simulink model "main"  (R2022a)
settings: Solver=FixedStepDiscrete  StartTime=0.0  StopTime=Inf  FixedStep=(50e-6)-(sim_en*4.995e-5)  RelTol=1e-3  EnableMultiTasking=on
model workspace (MAT data in the model file):
  Param : Simulink.Parameter (value not decoded)
  ac_ok : Simulink.Signal (value not decoded)
  ac_ok_120 : Simulink.Signal (value not decoded)
  bulk_voltage : Simulink.Signal (value not decoded)
  burstduty_integ_max : Simulink.Signal (value not decoded)
  burstduty_integ_min : Simulink.Signal (value not decoded)
  burstduty_ki : Simulink.Signal (value not decoded)
  burstduty_kp : Simulink.Signal (value not decoded)
  calib_ok : Simulink.Signal (value not decoded)
  can_addr1 : Simulink.Signal (value not decoded)
  can_addr2 : Simulink.Signal (value not decoded)
  can_addr3 : Simulink.Signal (value not decoded)
  can_addr4 : Simulink.Signal (value not decoded)
  can_data_rx : Simulink.Signal (value not decoded)
  can_data_tx : Simulink.Signal (value not decoded)
  can_timeout_120 : Simulink.Signal (value not decoded)
  chksum_scircv : Simulink.Signal (value not decoded)
  clllc_en_120 : Simulink.Signal (value not decoded)
  clllc_fault_120 : Simulink.Signal (value not decoded)
  clllc_ok_120 : Simulink.Signal (value not decoded)
  cmpss1h : Simulink.Signal (value not decoded)
  cmpss1l : Simulink.Signal (value not decoded)
  cmpss2h : Simulink.Signal (value not decoded)
  cmpss2l : Simulink.Signal (value not decoded)
  cmpss3h : Simulink.Signal (value not decoded)
  cmpss3l : Simulink.Signal (value not decoded)
  cmpss4h : Simulink.Signal (value not decoded)
  cmpss4l : Simulink.Signal (value not decoded)
  cmpss5h : Simulink.Signal (value not decoded)
  cmpss5l : Simulink.Signal (value not decoded)
  cmpss6h : Simulink.Signal (value not decoded)
  cmpss6l : Simulink.Signal (value not decoded)
  cmpss7h : Simulink.Signal (value not decoded)
  cmpss7l : Simulink.Signal (value not decoded)
  cmpss8h : Simulink.Signal (value not decoded)
  cmpss8l : Simulink.Signal (value not decoded)
  cnt_idle : Simulink.Signal (value not decoded)
  cnt_orps : Simulink.Signal (value not decoded)
  cnt_scircv : Simulink.Signal (value not decoded)
  cnt_scixmt : Simulink.Signal (value not decoded)
  cnt_scixmt_func : Simulink.Signal (value not decoded)
  cnt_temp_mux : Simulink.Signal (value not decoded)
  cnt_vdroop : Simulink.Signal (value not decoded)
  config_ok : Simulink.Signal (value not decoded)
  control_en : Simulink.Signal (value not decoded)
  cp_ready_120 : Simulink.Signal (value not decoded)
  d2d_en : Simulink.Signal (value not decoded)
  dchg_off : Simulink.Signal (value not decoded)
  debug_dacb : Simulink.Signal (value not decoded)
  debug_dacc : Simulink.Signal (value not decoded)
  debug_msg1 : Simulink.Signal (value not decoded)
  debug_msg2 : Simulink.Signal (value not decoded)
  debug_msg3 : Simulink.Signal (value not decoded)
  debug_msg4 : Simulink.Signal (value not decoded)
  debug_msg5 : Simulink.Signal (value not decoded)
  debug_msg6 : Simulink.Signal (value not decoded)
  dir_v2g : Simulink.Signal (value not decoded)
  eoss_llc1 : Simulink.Signal (value not decoded)
  eoss_llc2 : Simulink.Signal (value not decoded)
  eoss_orps : Simulink.Signal (value not decoded)
  fault_ocp : Simulink.Signal (value not decoded)
  fault_otp : Simulink.Signal (value not decoded)
  fault_ovp : Simulink.Signal (value not decoded)
  fut_en : Simulink.Signal (value not decoded)
  fwd_en_120 : Simulink.Signal (value not decoded)
  gain_llc1_sec_idc : Simulink.Signal (value not decoded)
  gain_llc1_temp_sr : Simulink.Signal (value not decoded)
  gain_llc2_sec_idc : Simulink.Signal (value not decoded)
  gain_vbat : Simulink.Signal (value not decoded)
  gain_vbulk : Simulink.Signal (value not decoded)
  gain_vout : Simulink.Signal (value not decoded)
  input_current_phasea : Simulink.Signal (value not decoded)
  input_current_phaseb : Simulink.Signal (value not decoded)
  input_current_phasec : Simulink.Signal (value not decoded)
  input_freq : Simulink.Signal (value not decoded)
  input_power : Simulink.Signal (value not decoded)
  input_voltage_phasea : Simulink.Signal (value not decoded)
  input_voltage_phaseb : Simulink.Signal (value not decoded)
  input_voltage_phasec : Simulink.Signal (value not decoded)
  ishare_arbiter : Simulink.Signal (value not decoded)
  ishare_thresh : Simulink.Signal (value not decoded)
  led_g : Simulink.Signal (value not decoded)
  led_r : Simulink.Signal (value not decoded)
  led_y : Simulink.Signal (value not decoded)
  llc1_burst_integ : Simulink.Signal (value not decoded)
  llc1_burstduty_buffer : Simulink.Signal (value not decoded)
  llc1_pfm_error : Simulink.Signal (value not decoded)
  llc1_pfm_integ : Simulink.Signal (value not decoded)
  llc1_pfm_prop : Simulink.Signal (value not decoded)
  llc1_pri_idc : Simulink.Signal (value not decoded)
  llc1_ps_buffer : Simulink.Signal (value not decoded)
  llc1_pspwm_error : Simulink.Signal (value not decoded)
  llc1_pspwm_integ : Simulink.Signal (value not decoded)
  llc1_pspwm_prop : Simulink.Signal (value not decoded)
  llc1_sec_idc : Simulink.Signal (value not decoded)
  llc1_temp_sr : Simulink.Signal (value not decoded)
  llc1_ts_tbctr_buffer : Simulink.Signal (value not decoded)
  llc2_burst_integ : Simulink.Signal (value not decoded)
  llc2_burstduty_buffer : Simulink.Signal (value not decoded)
  llc2_en : Simulink.Signal (value not decoded)
  llc2_en_buffer : Simulink.Signal (value not decoded)
  llc2_pfm_error : Simulink.Signal (value not decoded)
  llc2_pfm_integ : Simulink.Signal (value not decoded)
  llc2_pfm_prop : Simulink.Signal (value not decoded)
  llc2_pri_idc : Simulink.Signal (value not decoded)
  llc2_ps_buffer : Simulink.Signal (value not decoded)
  llc2_pspwm_error : Simulink.Signal (value not decoded)
  llc2_pspwm_integ : Simulink.Signal (value not decoded)
  llc2_pspwm_prop : Simulink.Signal (value not decoded)
  llc2_sec_idc : Simulink.Signal (value not decoded)
  llc2_temp_sr : Simulink.Signal (value not decoded)
  llc2_ts_tbctr_buffer : Simulink.Signal (value not decoded)
  loop_adcint : Simulink.Signal (value not decoded)
  loop_control : Simulink.Signal (value not decoded)
  loop_idle : Simulink.Signal (value not decoded)
  mid_bulk_voltage : Simulink.Signal (value not decoded)
  mode_120 : Simulink.Signal (value not decoded)
  mode_cc_cv : Simulink.Signal (value not decoded)
  myParam : mpt.Parameter (value not decoded)
  obc_ok_120 : Simulink.Signal (value not decoded)
  offset_llc1_sec_idc : Simulink.Signal (value not decoded)
  offset_llc1_temp_sr : Simulink.Signal (value not decoded)
  offset_llc2_sec_idc : Simulink.Signal (value not decoded)
  offset_vbat : Simulink.Signal (value not decoded)
  offset_vbulk : Simulink.Signal (value not decoded)
  offset_vout : Simulink.Signal (value not decoded)
  openloop_en : Simulink.Signal (value not decoded)
  openloop_fault_en : Simulink.Signal (value not decoded)
  ot_fault_120 : Simulink.Signal (value not decoded)
  pfc_en : Simulink.Signal (value not decoded)
  pfc_en_120 : Simulink.Signal (value not decoded)
  pfc_fw_revision : Simulink.Signal (value not decoded)
  pfc_fw_revision_bootloader : Simulink.Signal (value not decoded)
  pfc_fw_revision_debug : Simulink.Signal (value not decoded)
  pfc_ok : Simulink.Signal (value not decoded)
  pfc_ok_120 : Simulink.Signal (value not decoded)
  pfm_a0 : Simulink.Signal (value not decoded)
  pfm_a1 : Simulink.Signal (value not decoded)
  pfm_integ_max : Simulink.Signal (value not decoded)
  pfm_integ_min : Simulink.Signal (value not decoded)
  pfm_ki : Simulink.Signal (value not decoded)
  pfm_kp : Simulink.Signal (value not decoded)
  pri_fut_en : Simulink.Signal (value not decoded)
  pri_fut_en_buffer : Simulink.Signal (value not decoded)
  pri_halfbridge_en : Simulink.Signal (value not decoded)
  pri_halfbridge_en_buffer : Simulink.Signal (value not decoded)
  pspwm_integ_max : Simulink.Signal (value not decoded)
  pspwm_integ_min : Simulink.Signal (value not decoded)
  pspwm_ki : Simulink.Signal (value not decoded)
  pspwm_kp : Simulink.Signal (value not decoded)
  ref_idclink_max : Simulink.Signal (value not decoded)
  ref_iout : Simulink.Signal (value not decoded)
  ref_iout_calib : Simulink.Signal (value not decoded)
  ref_iout_llc1 : Simulink.Signal (value not decoded)
  ref_iout_llc1_calib : Simulink.Signal (value not decoded)
  ref_iout_llc2 : Simulink.Signal (value not decoded)
  ref_iout_llc2_calib : Simulink.Signal (value not decoded)
  ref_pout : Simulink.Signal (value not decoded)
  ref_ss_llc1 : Simulink.Signal (value not decoded)
  ref_ss_llc2 : Simulink.Signal (value not decoded)
  ref_ss_orps : Simulink.Signal (value not decoded)
  ref_vbat : Simulink.Signal (value not decoded)
  ref_vbat_calib : Simulink.Signal (value not decoded)
  ref_vbulk : Simulink.Signal (value not decoded)
  ref_vbulk_calib : Simulink.Signal (value not decoded)
  ref_vbulk_llc1_calib : Simulink.Signal (value not decoded)
  ref_vbulk_llc2_calib : Simulink.Signal (value not decoded)
  ref_vout : Simulink.Signal (value not decoded)
  ref_vout_calib : Simulink.Signal (value not decoded)
  relay_en : Simulink.Signal (value not decoded)
  reset_flag : Simulink.Signal (value not decoded)
  rev_en_120 : Simulink.Signal (value not decoded)
  runtime_control : Simulink.Signal (value not decoded)
  runtime_idle : Simulink.Signal (value not decoded)
  scircv_buffer : Simulink.Signal (value not decoded)
  scircv_buffer_tmp : Simulink.Signal (value not decoded)
  scircv_buffer_tmp_idx0 : Simulink.Signal (value not decoded)
  scircv_chksum : Simulink.Signal (value not decoded)
  scircv_chksum_ok : Simulink.Signal (value not decoded)
  scircv_parse_ok : Simulink.Signal (value not decoded)
  scixmt_buffer : Simulink.Signal (value not decoded)
  scixmt_chksum : Simulink.Signal (value not decoded)
  scixmt_func : Simulink.Signal (value not decoded)
  scixmt_word0_lsb : Simulink.Signal (value not decoded)
  scixmt_word0_msb : Simulink.Signal (value not decoded)
  scixmt_word1_lsb : Simulink.Signal (value not decoded)
  scixmt_word1_msb : Simulink.Signal (value not decoded)
  scixmt_word2_lsb : Simulink.Signal (value not decoded)
  scixmt_word2_msb : Simulink.Signal (value not decoded)
  scixmt_wr : Simulink.Signal (value not decoded)
  ss_step : Simulink.Signal (value not decoded)
  state_calib : Simulink.Signal (value not decoded)
  state_control : Simulink.Signal (value not decoded)
  state_hkeep : Simulink.Signal (value not decoded)
  status_cmpss : Simulink.Signal (value not decoded)
  status_control : Simulink.Signal (value not decoded)
  status_digin : Simulink.Signal (value not decoded)
  status_digout : Simulink.Signal (value not decoded)
  status_fault : Simulink.Signal (value not decoded)
  status_input : Simulink.Signal (value not decoded)
  status_pfc : Simulink.Signal (value not decoded)
  temp_inlet : Simulink.Signal (value not decoded)
  temp_llc1_fet_hs : Simulink.Signal (value not decoded)
  temp_llc2_fet_hs : Simulink.Signal (value not decoded)
  temp_mux : Simulink.Signal (value not decoded)
  temp_mux_s0 : Simulink.Signal (value not decoded)
  temp_mux_s1 : Simulink.Signal (value not decoded)
  temp_mux_s2 : Simulink.Signal (value not decoded)
  temp_outlet : Simulink.Signal (value not decoded)
  temp_pfc_fet_hsa : Simulink.Signal (value not decoded)
  temp_pfc_fet_hsb : Simulink.Signal (value not decoded)
  temp_pfc_fet_hsc : Simulink.Signal (value not decoded)
  temp_pfc_fet_lsa : Simulink.Signal (value not decoded)
  temp_pfc_fet_lsb : Simulink.Signal (value not decoded)
  temp_pfc_fet_lsc : Simulink.Signal (value not decoded)
  test_mode : Simulink.Signal (value not decoded)
  tfcv_cc : Simulink.Signal (value not decoded)
  tfcv_cc_llc2 : Simulink.Signal (value not decoded)
  tfcv_cv : Simulink.Signal (value not decoded)
  tfcv_sr_en : Simulink.Signal (value not decoded)
  tfv_assert_llc1_pri_idc : Simulink.Signal (value not decoded)
  tfv_assert_llc1_sec_idc : Simulink.Signal (value not decoded)
  tfv_assert_llc1_temp_sr : Simulink.Signal (value not decoded)
  tfv_assert_llc2_pri_idc : Simulink.Signal (value not decoded)
  tfv_assert_llc2_sec_idc : Simulink.Signal (value not decoded)
  tfv_assert_llc2_temp_sr : Simulink.Signal (value not decoded)
  tfv_assert_temp_outlet : Simulink.Signal (value not decoded)
  tfv_assert_vaux_uv : Simulink.Signal (value not decoded)
  tfv_assert_vbat : Simulink.Signal (value not decoded)
  tfv_assert_vbulk : Simulink.Signal (value not decoded)
  tfv_assert_vout : Simulink.Signal (value not decoded)
  tfv_cnt_tz : Simulink.Signal (value not decoded)
  tfv_deassert_llc1_pri_idc : Simulink.Signal (value not decoded)
  tfv_deassert_llc1_sec_idc : Simulink.Signal (value not decoded)
  tfv_deassert_llc1_temp_sr : Simulink.Signal (value not decoded)
  tfv_deassert_llc2_pri_idc : Simulink.Signal (value not decoded)
  tfv_deassert_llc2_sec_idc : Simulink.Signal (value not decoded)
  tfv_deassert_llc2_temp_sr : Simulink.Signal (value not decoded)
  tfv_deassert_temp_outlet : Simulink.Signal (value not decoded)
  tfv_deassert_vaux_uv : Simulink.Signal (value not decoded)
  tfv_deassert_vbat : Simulink.Signal (value not decoded)
  tfv_deassert_vbulk : Simulink.Signal (value not decoded)
  tfv_deassert_vout : Simulink.Signal (value not decoded)
  tfv_llc1_pri_idc : Simulink.Signal (value not decoded)
  tfv_llc1_sec_idc : Simulink.Signal (value not decoded)
  tfv_llc1_temp_sr : Simulink.Signal (value not decoded)
  tfv_llc2_pri_idc : Simulink.Signal (value not decoded)
  tfv_llc2_sec_idc : Simulink.Signal (value not decoded)
  tfv_llc2_temp_sr : Simulink.Signal (value not decoded)
  tfv_temp_outlet : Simulink.Signal (value not decoded)
  tfv_vaux_uv : Simulink.Signal (value not decoded)
  tfv_vbat : Simulink.Signal (value not decoded)
  tfv_vbulk : Simulink.Signal (value not decoded)
  tfv_vout : Simulink.Signal (value not decoded)
  timer_1ms : Simulink.Signal (value not decoded)
  tz : Simulink.Signal (value not decoded)
  valve_en : Simulink.Signal (value not decoded)
  vaux : Simulink.Signal (value not decoded)
  vbat : Simulink.Signal (value not decoded)
  vbulk : Simulink.Signal (value not decoded)
  vout : Simulink.Signal (value not decoded)
undefined symbols (not defined in the file or in its folder): CAN_O_INT, CANA_BASE, Down, GPTRIP1SEL, GPTRIP2SEL, TZ1, TZ2, Up
libraries: hdlsllib x159, simulink x100, c2837xDlib x24, c2807xlib x16, c280xlib x13, c2802xlib x12, canmsglib x8, idelinklib_common x2, c2000lib x1, c281xlib x1
(part 8 of 15)

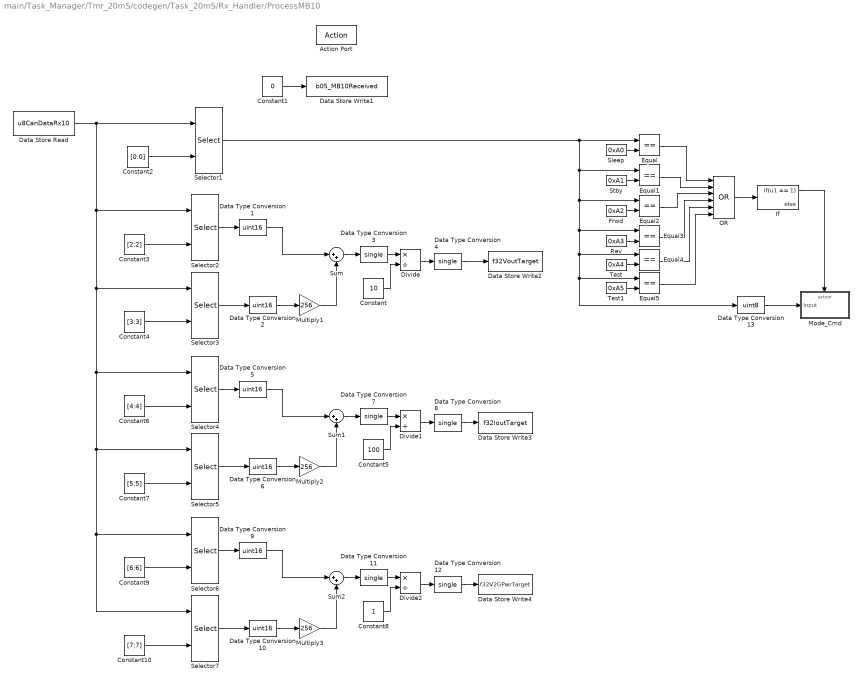
== system main/Task_Manager/Tmr_20mS/codegen/Task_20mS/Rx_Handler/ProcessMB10 ==
  Action Port : ActionPort  ActionPortLabel=if(u1 == 1)
  Constant : Constant  Value=10
  Constant1 : Constant  Value=0  OutDataTypeStr=boolean
  Constant10 : Constant  Value=[7:7]
  Constant2 : Constant  Value=[0:0]
  Constant3 : Constant  Value=[2:2]
  Constant4 : Constant  Value=[3:3]
  Constant5 : Constant  Value=100
  Constant6 : Constant  Value=[4:4]
  Constant7 : Constant  Value=[5:5]
  Constant8 : Constant
  Constant9 : Constant  Value=[6:6]
  Data Store Read : DataStoreRead  DataStoreName=u8CanDataRx10  IndexOptions=Index vector (dialog)  Indices=1  OutputSizes=1
  Data Store Write1 : DataStoreWrite  DataStoreName=b05_MB10Received  IndexOptions=Index vector (dialog)  Indices=1  OutputSizes=1
  Data Store Write2 : DataStoreWrite  DataStoreName=f32VoutTarget  IndexOptions=Index vector (dialog)  Indices=1  OutputSizes=1
  Data Store Write3 : DataStoreWrite  DataStoreName=f32IoutTarget  IndexOptions=Index vector (dialog)  Indices=1  OutputSizes=1
  Data Store Write4 : DataStoreWrite  DataStoreName=f32V2GPwrTarget  IndexOptions=Index vector (dialog)  Indices=1  OutputSizes=1
  Data Type Conversion{1..2,5..6,9..10} (6 alike) : DataTypeConversion  OutDataTypeStr=uint16  SaturateOnIntegerOverflow=off  RndMeth=Floor
  Data Type Conversion{3..4,7..8,11..12} (6 alike) : DataTypeConversion  OutDataTypeStr=single  SaturateOnIntegerOverflow=off  RndMeth=Floor
  Data Type Conversion13 : DataTypeConversion  OutDataTypeStr=uint8  SaturateOnIntegerOverflow=off  RndMeth=Floor
  Divide : Product  Inputs=*/
  Divide1 : Product  Inputs=*/
  Divide2 : Product  Inputs=*/
  Equal{,1..5} (6 alike) : RelationalOperator  Operator===  OutDataTypeStr=boolean  RndMeth=Simplest  InputSameDT=off
  Frwd : Constant  Value=0xA2
  If : If  IfExpression=u1 == 1
  Mode_Cmd : Subsystem  TreatAsAtomicUnit=on
  Multiply1 : Gain  Gain=256
  Multiply2 : Gain  Gain=256
  Multiply3 : Gain  Gain=256
  OR : Logic  Operator=OR  Inputs=6  IconShape=distinctive  AllPortsSameDT=off  OutDataTypeStr=boolean
  Rev : Constant  Value=0xA3
  Selector{1..7} (7 alike) : Selector  IndexMode=Zero-based  InputPortWidth=8  IndexOptions=Index vector (port)  Indices=[1 3]  OutputSizes=1
  Sleep : Constant  Value=0xA0
  Stby : Constant  Value=0xA1
  Sum : Sum  Inputs=|++
  Sum1 : Sum  Inputs=|++
  Sum2 : Sum  Inputs=|++
  Test : Constant  Value=0xA4
  Test1 : Constant  Value=0xA5
  wires:
  Constant1/1 -> Data Store Write1/1
  Constant2/1 -> Selector1/2
  Constant3/1 -> Selector2/2
  Constant4/1 -> Selector3/2
  Selector2/1 -> Data Type Conversion1/1
  Data Type Conversion1/1 -> Sum/1
  Selector3/1 -> Data Type Conversion2/1
  Data Type Conversion2/1 -> Multiply1/1
  Multiply1/1 -> Sum/2
  Sum/1 -> Data Type Conversion3/1
  Constant/1 -> Divide/2
  Divide/1 -> Data Type Conversion4/1
  Data Type Conversion3/1 -> Divide/1
  Data Type Conversion4/1 -> Data Store Write2/1
  Data Type Conversion8/1 -> Data Store Write3/1
  Data Type Conversion7/1 -> Divide1/1
  Divide1/1 -> Data Type Conversion8/1
  Constant5/1 -> Divide1/2
  Sum1/1 -> Data Type Conversion7/1
  Multiply2/1 -> Sum1/2
  Data Type Conversion6/1 -> Multiply2/1
  Selector5/1 -> Data Type Conversion6/1
  Data Type Conversion5/1 -> Sum1/1
  Selector4/1 -> Data Type Conversion5/1
  Constant7/1 -> Selector5/2
  Constant6/1 -> Selector4/2
  Constant9/1 -> Selector6/2
  Data Store Read/1 -> Selector6/1, Selector7/1, Selector5/1, Selector4/1, Selector3/1, Selector2/1, Selector1/1
  Constant10/1 -> Selector7/2
  Selector6/1 -> Data Type Conversion9/1
  Data Type Conversion9/1 -> Sum2/1
  Selector7/1 -> Data Type Conversion10/1
  Data Type Conversion10/1 -> Multiply3/1
  Multiply3/1 -> Sum2/2
  Sum2/1 -> Data Type Conversion11/1
  Constant8/1 -> Divide2/2
  Divide2/1 -> Data Type Conversion12/1
  Data Type Conversion11/1 -> Divide2/1
  Data Type Conversion12/1 -> Data Store Write4/1
  Stby/1 -> Equal1/2
  OR/1 -> If/1
  Rev/1 -> Equal3/2
  Equal1/1 -> OR/2
  Frwd/1 -> Equal2/2
  Equal2/1 -> OR/3
  Equal3/1 -> OR/4
  Data Type Conversion13/1 -> Mode_Cmd/1(Input)
  Equal/1 -> OR/1
  Sleep/1 -> Equal/2
  If/1 -> Mode_Cmd/Action
  Equal4/1 -> OR/5
  Selector1/1 -> Equal4/1, Data Type Conversion13/1, Equal5/1, Equal3/1, Equal2/1, Equal1/1, Equal/1
  Test/1 -> Equal4/2
  Equal5/1 -> OR/6
  Test1/1 -> Equal5/2

== system main/Task_Manager/Tmr_20mS/codegen/Task_20mS/Rx_Handler/ProcessMB11 ==
  Action Port : ActionPort  ActionPortLabel=elseif(u2 ==1)
  Constant : Constant  Value=0  OutDataTypeStr=boolean
  Constant1 : Constant  Value=[1:1]
  Constant2 : Constant  Value=[0:0]
  Data Store Read : DataStoreRead  DataStoreName=u8CanDataRx11  IndexOptions=Index vector (dialog)  Indices=1  OutputSizes=1
  Data Store Write1 : DataStoreWrite  DataStoreName=b06_MB11Received  IndexOptions=Index vector (dialog)  Indices=1  OutputSizes=1
  Data Store Write5 : DataStoreWrite  DataStoreName=u8AliveCounter  IndexOptions=Index vector (dialog)  Indices=1  OutputSizes=1
  Data Type Conversion : DataTypeConversion  OutDataTypeStr=uint8  SaturateOnIntegerOverflow=off  RndMeth=Floor
  Data Type Conversion1 : DataTypeConversion  OutDataTypeStr=uint8  SaturateOnIntegerOverflow=off  RndMeth=Floor
  Equal{,1..3} (4 alike) : RelationalOperator  Operator===  OutDataTypeStr=boolean  RndMeth=Simplest  InputSameDT=off
  If : If  IfExpression=u1 == 1
  OR : Logic  Operator=OR  Inputs=4  IconShape=distinctive  AllPortsSameDT=off  OutDataTypeStr=boolean
  Red_Frwd : Constant  Value=0xB2
  Red_Mode_Cmd : Subsystem  TreatAsAtomicUnit=on
  Red_Rev : Constant  Value=0xB3
  Red_Sleep : Constant  Value=0xB0
  Red_Stby : Constant  Value=0xB1
  Selector1 : Selector  IndexMode=Zero-based  InputPortWidth=8  IndexOptions=Index vector (port)  Indices=[1 3]  OutputSizes=1
  Selector2 : Selector  IndexMode=Zero-based  InputPortWidth=8  IndexOptions=Index vector (port)  Indices=[1 3]  OutputSizes=1
  wires:
  Constant/1 -> Data Store Write1/1
  Constant2/1 -> Selector1/2
  Data Type Conversion/1 -> Data Store Write5/1
  Selector1/1 -> Data Type Conversion/1
  Data Store Read/1 -> Selector2/1, Selector1/1
  Constant1/1 -> Selector2/2
  Red_Stby/1 -> Equal1/2
  Selector2/1 -> Equal/1, Data Type Conversion1/1, Equal3/1, Equal2/1, Equal1/1
  Equal2/1 -> OR/3
  Equal/1 -> OR/1
  If/1 -> Red_Mode_Cmd/Action
  OR/1 -> If/1
  Equal3/1 -> OR/4
  Equal1/1 -> OR/2
  Red_Rev/1 -> Equal3/2
  Red_Sleep/1 -> Equal/2
  Red_Frwd/1 -> Equal2/2
  Data Type Conversion1/1 -> Red_Mode_Cmd/1(Input)

== system main/Task_Manager/Tmr_20mS/codegen/Task_20mS/Rx_Handler/ProcessMB12 ==
  Action Port : ActionPort  ActionPortLabel=elseif( u3==1)
  Constant : Constant  Value=0  OutDataTypeStr=boolean
  Constant2 : Constant  Value=[0:0]
  Data Store Read : DataStoreRead  DataStoreName=u8CanDataRx12  IndexOptions=Index vector (dialog)  Indices=1  OutputSizes=1
  Data Store Write1 : DataStoreWrite  DataStoreName=b07_MB12Received  IndexOptions=Index vector (dialog)  Indices=1  OutputSizes=1
  Debug_Cmd : Subsystem  TreatAsAtomicUnit=on
  Debug_Read : Subsystem  TreatAsAtomicUnit=on
  Debug_Write : Subsystem  TreatAsAtomicUnit=on
  If : If  IfExpression=u1 == 0  ElseIfExpressions=u1 ==1, u1==2
  Selector1 : Selector  IndexMode=Zero-based  InputPortWidth=8  IndexOptions=Index vector (port)  Indices=[1 3]  OutputSizes=1
  wires:
  Constant/1 -> Data Store Write1/1
  Constant2/1 -> Selector1/2
  Data Store Read/1 -> Selector1/1
  Selector1/1 -> If/1
  If/1 -> Debug_Read/Action
  If/2 -> Debug_Write/Action
  If/3 -> Debug_Cmd/Action

== system main/Task_Manager/Tmr_20mS/codegen/Task_20mS/Tx_Handler/Run Tx Routine ==
  Action Port : ActionPort  ActionPortLabel=if(u1 == u2)
  Constant1 : Constant  Value=0  OutDataTypeStr=uint16
  Data Store Read2 : DataStoreRead  DataStoreName=b01_ReadRequest  IndexOptions=Index vector (dialog)  Indices=1  OutputSizes=1
  Data Store Read3 : DataStoreRead  DataStoreName=b00_DebugEnabled  IndexOptions=Index vector (dialog)  Indices=1  OutputSizes=1
  Data Store Write1 : DataStoreWrite  DataStoreName=u16TxDelayCount  IndexOptions=Index vector (dialog)  Indices=1  OutputSizes=1
  If1 : If  NumInputs=2  IfExpression=u1 == 1 & u2 == 1
  TxReadRequest : Subsystem  TreatAsAtomicUnit=on
  TxStatusData : Subsystem  TreatAsAtomicUnit=on
  wires:
  Constant1/1 -> Data Store Write1/1
  If1/1 -> TxReadRequest/Action
  If1/2 -> TxStatusData/Action
  Data Store Read3/1 -> If1/2
  Data Store Read2/1 -> If1/1

== system main/Task_Manager/idle/idle_task/comm_npc/comm_npc/COMM_NPC.calcScircvChksum/For Iterator Subsystem ==
  scircv_buffer : Inport
  Bitwise XOR : simulink/Logic and Bit Operations/Bitwise Operator  logicop=XOR  UseBitMask=off  NumInputPorts=2  BitMask=bin2dec('11011001')  BitMaskRealWorld=Stored Integer
  Data Store Read1 : DataStoreRead  DataStoreName=scircv_chksum  IndexOptions=Index vector (dialog)  Indices=1  OutputSizes=1
  Data Store Write : DataStoreWrite  DataStoreName=scircv_chksum  IndexOptions=Index vector (dialog)  Indices=1  OutputSizes=1
  For Iterator : ForIterator  IterationLimit=9  IndexMode=Zero-based  IterationVariableDataType=uint8
  Selector : Selector  IndexMode=Zero-based  InputPortWidth=12  IndexOptions=Index vector (port)  Indices=[1 3]  OutputSizes=1
  wires:
  For Iterator/1 -> Selector/2
  scircv_buffer/1 -> Selector/1
  Selector/1 -> Bitwise XOR/1
  Data Store Read1/1 -> Bitwise XOR/2
  Bitwise XOR/1 -> Data Store Write/1

== system main/Task_Manager/idle/idle_task/comm_npc/comm_npc/COMM_NPC.calcScixmtChksum/calc_chksum ==
  function : TriggerPort  TriggerType=function-call  VariantControl=Variant
  Data Store Read8 : DataStoreRead  DataStoreName=scixmt_buffer  IndexOptions=Index vector (dialog)  Indices=1  OutputSizes=1
  For Iterator Subsystem : Subsystem  TreatAsAtomicUnit=on
  wires:
  Data Store Read8/1 -> For Iterator Subsystem/1(scixmt_buffer)

== system main/Task_Manager/idle/idle_task/comm_npc/comm_npc/COMM_NPC.calcScixmtChksum/update_scixmt_buffer ==
  function : TriggerPort  TriggerType=function-call  VariantControl=Variant
  Data Store Read21 : DataStoreRead  DataStoreName=scixmt_func  IndexOptions=Index vector (dialog)  Indices=1  OutputSizes=1
  If : If  IfExpression=u1 == 33
  default : Subsystem  TreatAsAtomicUnit=on
  pri_fut_en : Subsystem  TreatAsAtomicUnit=on
  wires:
  If/1 -> pri_fut_en/Action
  If/2 -> default/Action
  Data Store Read21/1 -> default/1(scixmt_func), If/1

== system main/Task_Manager/idle/idle_task/comm_npc/comm_npc/COMM_NPC.extractScircv/input_main_info ==
  note: Note:
      | byte0 - header
      | byte1 - w/r
      | byte2 - func
      | byte3, byte4 - word0_lsb, word0_msb
      | byte5, byte6 - word1_lsb, word1_msb
      | byte7, byte8 - word2_lsb, word2_msb
      | byte9 - chksum
      | byte10 - 0x00
      | byte11 - terminator
  scircv_buffer : Inport
  Action Port : ActionPort  ActionPortLabel=case [ 1 ]:
  Add : Sum  AccumDataTypeStr=uint16  OutDataTypeStr=uint16
  Add1 : Sum  AccumDataTypeStr=uint16  OutDataTypeStr=uint16
  Add2 : Sum  AccumDataTypeStr=uint16  OutDataTypeStr=uint16
  Bit Shift : hdlsllib/Logic and Bit Operations/Bit Shift  mode=Shift Left Logical  N=8
  Bit Shift1 : hdlsllib/Logic and Bit Operations/Bit Shift  mode=Shift Left Logical  N=8
  Bit Shift2 : hdlsllib/Logic and Bit Operations/Bit Shift  mode=Shift Left Logical  N=8
  Cast To Single{1..6} (6 alike) : DataTypeConversion  OutDataTypeStr=uint16  SaturateOnIntegerOverflow=off  RndMeth=Floor
  Constant1 : Constant  Value=3  OutDataTypeStr=uint8
  Constant2 : Constant  Value=4  OutDataTypeStr=uint8
  Constant3 : Constant  Value=7  OutDataTypeStr=uint8
  Constant4 : Constant  Value=8  OutDataTypeStr=uint8
  Constant5 : Constant  Value=5  OutDataTypeStr=uint8
  Constant6 : Constant  Value=6  OutDataTypeStr=uint8
  Data Store Write1 : DataStoreWrite  DataStoreName=status_input  IndexOptions=Index vector (dialog)  Indices=1  OutputSizes=1
  Data Store Write2 : DataStoreWrite  DataStoreName=input_power  IndexOptions=Index vector (dialog)  Indices=1  OutputSizes=1
  Data Store Write3 : DataStoreWrite  DataStoreName=input_freq  IndexOptions=Index vector (dialog)  Indices=1  OutputSizes=1
  word0_lsb : Selector  IndexMode=Zero-based  InputPortWidth=12  IndexOptions=Index vector (port)  Indices=[1 3]  OutputSizes=1
  word0_lsb1 : Selector  IndexMode=Zero-based  InputPortWidth=12  IndexOptions=Index vector (port)  Indices=[1 3]  OutputSizes=1
  word0_lsb2 : Selector  IndexMode=Zero-based  InputPortWidth=12  IndexOptions=Index vector (port)  Indices=[1 3]  OutputSizes=1
  word0_msb : Selector  IndexMode=Zero-based  InputPortWidth=12  IndexOptions=Index vector (port)  Indices=[1 3]  OutputSizes=1
  word0_msb1 : Selector  IndexMode=Zero-based  InputPortWidth=12  IndexOptions=Index vector (port)  Indices=[1 3]  OutputSizes=1
  word0_msb2 : Selector  IndexMode=Zero-based  InputPortWidth=12  IndexOptions=Index vector (port)  Indices=[1 3]  OutputSizes=1
  wires:
  [scircv_buffer] -> word0_lsb2/1
  Constant5/1 -> word0_lsb2/2
  word0_lsb2/1 -> Cast To Single5/1
  Constant6/1 -> word0_msb2/2
  [scircv_buffer] -> word0_msb2/1
  word0_msb2/1 -> Cast To Single6/1
  Bit Shift2/1 -> Add2/2
  Add2/1 -> Data Store Write3/1
  Cast To Single5/1 -> Add2/1
  Cast To Single6/1 -> Bit Shift2/1
  [scircv_buffer] -> word0_lsb1/1
  Constant3/1 -> word0_lsb1/2
  word0_lsb1/1 -> Cast To Single3/1
  Constant4/1 -> word0_msb1/2
  [scircv_buffer] -> word0_msb1/1
  word0_msb1/1 -> Cast To Single4/1
  Bit Shift1/1 -> Add1/2
  Add1/1 -> Data Store Write2/1
  Cast To Single3/1 -> Add1/1
  Cast To Single4/1 -> Bit Shift1/1
  Cast To Single2/1 -> Bit Shift/1
  Cast To Single1/1 -> Add/1
  Add/1 -> Data Store Write1/1
  Bit Shift/1 -> Add/2
  word0_msb/1 -> Cast To Single2/1
  [scircv_buffer] -> word0_msb/1
  Constant2/1 -> word0_msb/2
  scircv_buffer/1 -> [scircv_buffer]
  word0_lsb/1 -> Cast To Single1/1
  Constant1/1 -> word0_lsb/2
  [scircv_buffer] -> word0_lsb/1

== system main/Task_Manager/idle/idle_task/comm_npc/comm_npc/COMM_NPC.extractScircv/input_phase_current ==
  note: Note:
      | byte0 - header
      | byte1 - w/r
      | byte2 - func
      | byte3, byte4 - word0_lsb, word0_msb
      | byte5, byte6 - word1_lsb, word1_msb
      | byte7, byte8 - word2_lsb, word2_msb
      | byte9 - chksum
      | byte10 - 0x00
      | byte11 - terminator
  scircv_buffer : Inport
  Action Port : ActionPort  ActionPortLabel=case [ 3 ]:
  Add : Sum  AccumDataTypeStr=uint16  OutDataTypeStr=uint16
  Add1 : Sum  AccumDataTypeStr=uint16  OutDataTypeStr=uint16
  Add2 : Sum  AccumDataTypeStr=uint16  OutDataTypeStr=uint16
  Bit Shift : hdlsllib/Logic and Bit Operations/Bit Shift  mode=Shift Left Logical  N=8
  Bit Shift1 : hdlsllib/Logic and Bit Operations/Bit Shift  mode=Shift Left Logical  N=8
  Bit Shift2 : hdlsllib/Logic and Bit Operations/Bit Shift  mode=Shift Left Logical  N=8
  Cast To Single{1..6} (6 alike) : DataTypeConversion  OutDataTypeStr=uint16  SaturateOnIntegerOverflow=off  RndMeth=Floor
  Constant1 : Constant  Value=3  OutDataTypeStr=uint8
  Constant2 : Constant  Value=4  OutDataTypeStr=uint8
  Constant3 : Constant  Value=7  OutDataTypeStr=uint8
  Constant4 : Constant  Value=8  OutDataTypeStr=uint8
  Constant5 : Constant  Value=5  OutDataTypeStr=uint8
  Constant6 : Constant  Value=6  OutDataTypeStr=uint8
  Data Store Write : DataStoreWrite  DataStoreName=input_current_phasea  IndexOptions=Index vector (dialog)  Indices=1  OutputSizes=1
  Data Store Write1 : DataStoreWrite  DataStoreName=input_current_phasea  IndexOptions=Index vector (dialog)  Indices=1  OutputSizes=1
  Data Store Write2 : DataStoreWrite  DataStoreName=input_current_phasec  IndexOptions=Index vector (dialog)  Indices=1  OutputSizes=1
  Data Store Write3 : DataStoreWrite  DataStoreName=input_current_phaseb  IndexOptions=Index vector (dialog)  Indices=1  OutputSizes=1
  Data Store Write4 : DataStoreWrite  DataStoreName=input_current_phaseb  IndexOptions=Index vector (dialog)  Indices=1  OutputSizes=1
  word0_lsb : Selector  IndexMode=Zero-based  InputPortWidth=12  IndexOptions=Index vector (port)  Indices=[1 3]  OutputSizes=1
  word0_lsb1 : Selector  IndexMode=Zero-based  InputPortWidth=12  IndexOptions=Index vector (port)  Indices=[1 3]  OutputSizes=1
  word0_lsb2 : Selector  IndexMode=Zero-based  InputPortWidth=12  IndexOptions=Index vector (port)  Indices=[1 3]  OutputSizes=1
  word0_msb : Selector  IndexMode=Zero-based  InputPortWidth=12  IndexOptions=Index vector (port)  Indices=[1 3]  OutputSizes=1
  word0_msb1 : Selector  IndexMode=Zero-based  InputPortWidth=12  IndexOptions=Index vector (port)  Indices=[1 3]  OutputSizes=1
  word0_msb2 : Selector  IndexMode=Zero-based  InputPortWidth=12  IndexOptions=Index vector (port)  Indices=[1 3]  OutputSizes=1
  wires:
  [scircv_buffer] -> word0_lsb2/1
  Constant5/1 -> word0_lsb2/2
  word0_lsb2/1 -> Cast To Single5/1
  Constant6/1 -> word0_msb2/2
  [scircv_buffer] -> word0_msb2/1
  word0_msb2/1 -> Cast To Single6/1
  Bit Shift2/1 -> Add2/2
  Add2/1 -> Data Store Write3/1
  Cast To Single5/1 -> Add2/1
  Cast To Single6/1 -> Bit Shift2/1
  [scircv_buffer] -> word0_lsb1/1
  Constant3/1 -> word0_lsb1/2
  word0_lsb1/1 -> Cast To Single3/1
  Constant4/1 -> word0_msb1/2
  [scircv_buffer] -> word0_msb1/1
  word0_msb1/1 -> Cast To Single4/1
  Bit Shift1/1 -> Add1/2
  Add1/1 -> Data Store Write2/1
  Cast To Single3/1 -> Add1/1
  Cast To Single4/1 -> Bit Shift1/1
  Cast To Single2/1 -> Bit Shift/1
  Cast To Single1/1 -> Add/1
  Add/1 -> Data Store Write1/1
  Bit Shift/1 -> Add/2
  word0_msb/1 -> Cast To Single2/1
  [scircv_buffer] -> word0_msb/1
  Constant2/1 -> word0_msb/2
  scircv_buffer/1 -> [scircv_buffer]
  word0_lsb/1 -> Cast To Single1/1
  Constant1/1 -> word0_lsb/2
  [scircv_buffer] -> word0_lsb/1

== system main/Task_Manager/idle/idle_task/comm_npc/comm_npc/COMM_NPC.extractScircv/input_phase_voltage ==
  note: Note:
      | byte0 - header
      | byte1 - w/r
      | byte2 - func
      | byte3, byte4 - word0_lsb, word0_msb
      | byte5, byte6 - word1_lsb, word1_msb
      | byte7, byte8 - word2_lsb, word2_msb
      | byte9 - chksum
      | byte10 - 0x00
      | byte11 - terminator
  scircv_buffer : Inport
  Action Port : ActionPort  ActionPortLabel=case [ 2 ]:
  Add : Sum  AccumDataTypeStr=uint16  OutDataTypeStr=uint16
  Add1 : Sum  AccumDataTypeStr=uint16  OutDataTypeStr=uint16
  Add2 : Sum  AccumDataTypeStr=uint16  OutDataTypeStr=uint16
  Bit Shift : hdlsllib/Logic and Bit Operations/Bit Shift  mode=Shift Left Logical  N=8
  Bit Shift1 : hdlsllib/Logic and Bit Operations/Bit Shift  mode=Shift Left Logical  N=8
  Bit Shift2 : hdlsllib/Logic and Bit Operations/Bit Shift  mode=Shift Left Logical  N=8
  Cast To Single{1..6} (6 alike) : DataTypeConversion  OutDataTypeStr=uint16  SaturateOnIntegerOverflow=off  RndMeth=Floor
  Constant1 : Constant  Value=3  OutDataTypeStr=uint8
  Constant2 : Constant  Value=4  OutDataTypeStr=uint8
  Constant3 : Constant  Value=7  OutDataTypeStr=uint8
  Constant4 : Constant  Value=8  OutDataTypeStr=uint8
  Constant5 : Constant  Value=5  OutDataTypeStr=uint8
  Constant6 : Constant  Value=6  OutDataTypeStr=uint8
  Data Store Write1 : DataStoreWrite  DataStoreName=input_voltage_phasea  IndexOptions=Index vector (dialog)  Indices=1  OutputSizes=1
  Data Store Write2 : DataStoreWrite  DataStoreName=input_voltage_phasec  IndexOptions=Index vector (dialog)  Indices=1  OutputSizes=1
  Data Store Write3 : DataStoreWrite  DataStoreName=input_voltage_phaseb  IndexOptions=Index vector (dialog)  Indices=1  OutputSizes=1
  word0_lsb : Selector  IndexMode=Zero-based  InputPortWidth=12  IndexOptions=Index vector (port)  Indices=[1 3]  OutputSizes=1
  word0_lsb1 : Selector  IndexMode=Zero-based  InputPortWidth=12  IndexOptions=Index vector (port)  Indices=[1 3]  OutputSizes=1
  word0_lsb2 : Selector  IndexMode=Zero-based  InputPortWidth=12  IndexOptions=Index vector (port)  Indices=[1 3]  OutputSizes=1
  word0_msb : Selector  IndexMode=Zero-based  InputPortWidth=12  IndexOptions=Index vector (port)  Indices=[1 3]  OutputSizes=1
  word0_msb1 : Selector  IndexMode=Zero-based  InputPortWidth=12  IndexOptions=Index vector (port)  Indices=[1 3]  OutputSizes=1
  word0_msb2 : Selector  IndexMode=Zero-based  InputPortWidth=12  IndexOptions=Index vector (port)  Indices=[1 3]  OutputSizes=1
  wires:
  [scircv_buffer] -> word0_lsb/1
  Constant1/1 -> word0_lsb/2
  word0_lsb/1 -> Cast To Single1/1
  scircv_buffer/1 -> [scircv_buffer]
  Constant2/1 -> word0_msb/2
  [scircv_buffer] -> word0_msb/1
  word0_msb/1 -> Cast To Single2/1
  Bit Shift/1 -> Add/2
  Add/1 -> Data Store Write1/1
  Cast To Single1/1 -> Add/1
  Cast To Single2/1 -> Bit Shift/1
  Cast To Single4/1 -> Bit Shift1/1
  Cast To Single3/1 -> Add1/1
  Add1/1 -> Data Store Write2/1
  Bit Shift1/1 -> Add1/2
  word0_msb1/1 -> Cast To Single4/1
  [scircv_buffer] -> word0_msb1/1
  Constant4/1 -> word0_msb1/2
  word0_lsb1/1 -> Cast To Single3/1
  Constant3/1 -> word0_lsb1/2
  [scircv_buffer] -> word0_lsb1/1
  Cast To Single6/1 -> Bit Shift2/1
  Cast To Single5/1 -> Add2/1
  Add2/1 -> Data Store Write3/1
  Bit Shift2/1 -> Add2/2
  word0_msb2/1 -> Cast To Single6/1
  [scircv_buffer] -> word0_msb2/1
  Constant6/1 -> word0_msb2/2
  word0_lsb2/1 -> Cast To Single5/1
  Constant5/1 -> word0_lsb2/2
  [scircv_buffer] -> word0_lsb2/1

== system main/Task_Manager/idle/idle_task/comm_npc/comm_npc/COMM_NPC.extractScircv/pfc_extra_info ==
  note: Note:
      | byte0 - header
      | byte1 - w/r
      | byte2 - func
      | byte3, byte4 - word0_lsb, word0_msb
      | byte5, byte6 - word1_lsb, word1_msb
      | byte7, byte8 - word2_lsb, word2_msb
      | byte9 - chksum
      | byte10 - 0x00
      | byte11 - terminator
  scircv_buffer : Inport
  Action Port : ActionPort  ActionPortLabel=case [ 5 ]:
  Add : Sum  AccumDataTypeStr=uint16  OutDataTypeStr=uint16
  Add1 : Sum  AccumDataTypeStr=uint16  OutDataTypeStr=uint16
  Add2 : Sum  AccumDataTypeStr=uint16  OutDataTypeStr=uint16
  Bit Shift : hdlsllib/Logic and Bit Operations/Bit Shift  mode=Shift Left Logical  N=8
  Bit Shift1 : hdlsllib/Logic and Bit Operations/Bit Shift  mode=Shift Left Logical  N=8
  Bit Shift2 : hdlsllib/Logic and Bit Operations/Bit Shift  mode=Shift Left Logical  N=8
  Cast To Single{1..6} (6 alike) : DataTypeConversion  OutDataTypeStr=uint16  SaturateOnIntegerOverflow=off  RndMeth=Floor
  Constant1 : Constant  Value=3  OutDataTypeStr=uint8
  Constant2 : Constant  Value=4  OutDataTypeStr=uint8
  Constant3 : Constant  Value=7  OutDataTypeStr=uint8
  Constant4 : Constant  Value=8  OutDataTypeStr=uint8
  Constant5 : Constant  Value=5  OutDataTypeStr=uint8
  Constant6 : Constant  Value=6  OutDataTypeStr=uint8
  Data Store Write1 : DataStoreWrite  DataStoreName=pfc_fw_revision_debug  IndexOptions=Index vector (dialog)  Indices=1  OutputSizes=1
  Data Store Write2 : DataStoreWrite  DataStoreName=pfc_fw_revision_bootloader  IndexOptions=Index vector (dialog)  Indices=1  OutputSizes=1
  Data Store Write3 : DataStoreWrite  DataStoreName=pfc_fw_revision  IndexOptions=Index vector (dialog)  Indices=1  OutputSizes=1
  word0_lsb : Selector  IndexMode=Zero-based  InputPortWidth=12  IndexOptions=Index vector (port)  Indices=[1 3]  OutputSizes=1
  word0_lsb1 : Selector  IndexMode=Zero-based  InputPortWidth=12  IndexOptions=Index vector (port)  Indices=[1 3]  OutputSizes=1
  word0_lsb2 : Selector  IndexMode=Zero-based  InputPortWidth=12  IndexOptions=Index vector (port)  Indices=[1 3]  OutputSizes=1
  word0_msb : Selector  IndexMode=Zero-based  InputPortWidth=12  IndexOptions=Index vector (port)  Indices=[1 3]  OutputSizes=1
  word0_msb1 : Selector  IndexMode=Zero-based  InputPortWidth=12  IndexOptions=Index vector (port)  Indices=[1 3]  OutputSizes=1
  word0_msb2 : Selector  IndexMode=Zero-based  InputPortWidth=12  IndexOptions=Index vector (port)  Indices=[1 3]  OutputSizes=1
  wires:
  [scircv_buffer] -> word0_lsb2/1
  Constant5/1 -> word0_lsb2/2
  word0_lsb2/1 -> Cast To Single5/1
  Constant6/1 -> word0_msb2/2
  [scircv_buffer] -> word0_msb2/1
  word0_msb2/1 -> Cast To Single6/1
  Bit Shift2/1 -> Add2/2
  Add2/1 -> Data Store Write3/1
  Cast To Single5/1 -> Add2/1
  Cast To Single6/1 -> Bit Shift2/1
  [scircv_buffer] -> word0_lsb1/1
  Constant3/1 -> word0_lsb1/2
  word0_lsb1/1 -> Cast To Single3/1
  Constant4/1 -> word0_msb1/2
  [scircv_buffer] -> word0_msb1/1
  word0_msb1/1 -> Cast To Single4/1
  Bit Shift1/1 -> Add1/2
  Add1/1 -> Data Store Write2/1
  Cast To Single3/1 -> Add1/1
  Cast To Single4/1 -> Bit Shift1/1
  Cast To Single2/1 -> Bit Shift/1
  Cast To Single1/1 -> Add/1
  Add/1 -> Data Store Write1/1
  Bit Shift/1 -> Add/2
  word0_msb/1 -> Cast To Single2/1
  [scircv_buffer] -> word0_msb/1
  Constant2/1 -> word0_msb/2
  scircv_buffer/1 -> [scircv_buffer]
  word0_lsb/1 -> Cast To Single1/1
  Constant1/1 -> word0_lsb/2
  [scircv_buffer] -> word0_lsb/1

== system main/Task_Manager/idle/idle_task/comm_npc/comm_npc/COMM_NPC.extractScircv/pfc_main_info ==
  note: Note:
      | byte0 - header
      | byte1 - w/r
      | byte2 - func
      | byte3, byte4 - word0_lsb, word0_msb
      | byte5, byte6 - word1_lsb, word1_msb
      | byte7, byte8 - word2_lsb, word2_msb
      | byte9 - chksum
      | byte10 - 0x00
      | byte11 - terminator
  scircv_buffer : Inport
  Action Port : ActionPort  ActionPortLabel=case [ 4 ]:
  Add : Sum  AccumDataTypeStr=uint16  OutDataTypeStr=uint16
  Add1 : Sum  AccumDataTypeStr=uint16  OutDataTypeStr=uint16
  Add2 : Sum  AccumDataTypeStr=uint16  OutDataTypeStr=uint16
  Bit Shift : hdlsllib/Logic and Bit Operations/Bit Shift  mode=Shift Left Logical  N=8
  Bit Shift1 : hdlsllib/Logic and Bit Operations/Bit Shift  mode=Shift Left Logical  N=8
  Bit Shift2 : hdlsllib/Logic and Bit Operations/Bit Shift  mode=Shift Left Logical  N=8
  Cast To Single{1..6} (6 alike) : DataTypeConversion  OutDataTypeStr=uint16  SaturateOnIntegerOverflow=off  RndMeth=Floor
  Constant1 : Constant  Value=3  OutDataTypeStr=uint8
  Constant2 : Constant  Value=4  OutDataTypeStr=uint8
  Constant3 : Constant  Value=7  OutDataTypeStr=uint8
  Constant4 : Constant  Value=8  OutDataTypeStr=uint8
  Constant5 : Constant  Value=5  OutDataTypeStr=uint8
  Constant6 : Constant  Value=6  OutDataTypeStr=uint8
  Data Store Write1 : DataStoreWrite  DataStoreName=status_pfc  IndexOptions=Index vector (dialog)  Indices=1  OutputSizes=1
  Data Store Write2 : DataStoreWrite  DataStoreName=mid_bulk_voltage  IndexOptions=Index vector (dialog)  Indices=1  OutputSizes=1
  Data Store Write3 : DataStoreWrite  DataStoreName=bulk_voltage  IndexOptions=Index vector (dialog)  Indices=1  OutputSizes=1
  word0_lsb : Selector  IndexMode=Zero-based  InputPortWidth=12  IndexOptions=Index vector (port)  Indices=[1 3]  OutputSizes=1
  word0_lsb1 : Selector  IndexMode=Zero-based  InputPortWidth=12  IndexOptions=Index vector (port)  Indices=[1 3]  OutputSizes=1
  word0_lsb2 : Selector  IndexMode=Zero-based  InputPortWidth=12  IndexOptions=Index vector (port)  Indices=[1 3]  OutputSizes=1
  word0_msb : Selector  IndexMode=Zero-based  InputPortWidth=12  IndexOptions=Index vector (port)  Indices=[1 3]  OutputSizes=1
  word0_msb1 : Selector  IndexMode=Zero-based  InputPortWidth=12  IndexOptions=Index vector (port)  Indices=[1 3]  OutputSizes=1
  word0_msb2 : Selector  IndexMode=Zero-based  InputPortWidth=12  IndexOptions=Index vector (port)  Indices=[1 3]  OutputSizes=1
  wires:
  [scircv_buffer] -> word0_lsb/1
  Constant1/1 -> word0_lsb/2
  word0_lsb/1 -> Cast To Single1/1
  scircv_buffer/1 -> [scircv_buffer]
  Constant2/1 -> word0_msb/2
  [scircv_buffer] -> word0_msb/1
  word0_msb/1 -> Cast To Single2/1
  Bit Shift/1 -> Add/2
  Add/1 -> Data Store Write1/1
  Cast To Single1/1 -> Add/1
  Cast To Single2/1 -> Bit Shift/1
  Cast To Single4/1 -> Bit Shift1/1
  Cast To Single3/1 -> Add1/1
  Add1/1 -> Data Store Write2/1
  Bit Shift1/1 -> Add1/2
  word0_msb1/1 -> Cast To Single4/1
  [scircv_buffer] -> word0_msb1/1
  Constant4/1 -> word0_msb1/2
  word0_lsb1/1 -> Cast To Single3/1
  Constant3/1 -> word0_lsb1/2
  [scircv_buffer] -> word0_lsb1/1
  Cast To Single6/1 -> Bit Shift2/1
  Cast To Single5/1 -> Add2/1
  Add2/1 -> Data Store Write3/1
  Bit Shift2/1 -> Add2/2
  word0_msb2/1 -> Cast To Single6/1
  [scircv_buffer] -> word0_msb2/1
  Constant6/1 -> word0_msb2/2
  word0_lsb2/1 -> Cast To Single5/1
  Constant5/1 -> word0_lsb2/2
  [scircv_buffer] -> word0_lsb2/1

== system main/Task_Manager/idle/idle_task/comm_npc/comm_npc/COMM_NPC.extractScircv/pri_debug_msga ==
  note: Note:
      | byte0 - header
      | byte1 - w/r
      | byte2 - func
      | byte3, byte4 - word0_lsb, word0_msb
      | byte5, byte6 - word1_lsb, word1_msb
      | byte7, byte8 - word2_lsb, word2_msb
      | byte9 - chksum
      | byte10 - 0x00
      | byte11 - terminator
  scircv_buffer : Inport
  Action Port : ActionPort  ActionPortLabel=case [ 49 ]:
  Add : Sum  AccumDataTypeStr=uint16  OutDataTypeStr=uint16
  Add1 : Sum  AccumDataTypeStr=uint16  OutDataTypeStr=uint16
  Add2 : Sum  AccumDataTypeStr=uint16  OutDataTypeStr=uint16
  Bit Shift : hdlsllib/Logic and Bit Operations/Bit Shift  mode=Shift Left Logical  N=8
  Bit Shift1 : hdlsllib/Logic and Bit Operations/Bit Shift  mode=Shift Left Logical  N=8
  Bit Shift2 : hdlsllib/Logic and Bit Operations/Bit Shift  mode=Shift Left Logical  N=8
  Cast To Single{1..6} (6 alike) : DataTypeConversion  OutDataTypeStr=uint16  SaturateOnIntegerOverflow=off  RndMeth=Floor
  Constant1 : Constant  Value=3  OutDataTypeStr=uint8
  Constant2 : Constant  Value=4  OutDataTypeStr=uint8
  Constant3 : Constant  Value=7  OutDataTypeStr=uint8
  Constant4 : Constant  Value=8  OutDataTypeStr=uint8
  Constant5 : Constant  Value=5  OutDataTypeStr=uint8
  Constant6 : Constant  Value=6  OutDataTypeStr=uint8
  Data Store Write1 : DataStoreWrite  DataStoreName=debug_msg1  IndexOptions=Index vector (dialog)  Indices=1  OutputSizes=1
  Data Store Write2 : DataStoreWrite  DataStoreName=debug_msg3  IndexOptions=Index vector (dialog)  Indices=1  OutputSizes=1
  Data Store Write3 : DataStoreWrite  DataStoreName=debug_msg2  IndexOptions=Index vector (dialog)  Indices=1  OutputSizes=1
  word0_lsb : Selector  IndexMode=Zero-based  InputPortWidth=12  IndexOptions=Index vector (port)  Indices=[1 3]  OutputSizes=1
  word0_lsb1 : Selector  IndexMode=Zero-based  InputPortWidth=12  IndexOptions=Index vector (port)  Indices=[1 3]  OutputSizes=1
  word0_lsb2 : Selector  IndexMode=Zero-based  InputPortWidth=12  IndexOptions=Index vector (port)  Indices=[1 3]  OutputSizes=1
  word0_msb : Selector  IndexMode=Zero-based  InputPortWidth=12  IndexOptions=Index vector (port)  Indices=[1 3]  OutputSizes=1
  word0_msb1 : Selector  IndexMode=Zero-based  InputPortWidth=12  IndexOptions=Index vector (port)  Indices=[1 3]  OutputSizes=1
  word0_msb2 : Selector  IndexMode=Zero-based  InputPortWidth=12  IndexOptions=Index vector (port)  Indices=[1 3]  OutputSizes=1
  wires:
  [scircv_buffer] -> word0_lsb2/1
  Constant5/1 -> word0_lsb2/2
  word0_lsb2/1 -> Cast To Single5/1
  Constant6/1 -> word0_msb2/2
  [scircv_buffer] -> word0_msb2/1
  word0_msb2/1 -> Cast To Single6/1
  Bit Shift2/1 -> Add2/2
  Add2/1 -> Data Store Write3/1
  Cast To Single5/1 -> Add2/1
  Cast To Single6/1 -> Bit Shift2/1
  [scircv_buffer] -> word0_lsb1/1
  Constant3/1 -> word0_lsb1/2
  word0_lsb1/1 -> Cast To Single3/1
  Constant4/1 -> word0_msb1/2
  [scircv_buffer] -> word0_msb1/1
  word0_msb1/1 -> Cast To Single4/1
  Bit Shift1/1 -> Add1/2
  Add1/1 -> Data Store Write2/1
  Cast To Single3/1 -> Add1/1
  Cast To Single4/1 -> Bit Shift1/1
  Cast To Single2/1 -> Bit Shift/1
  Cast To Single1/1 -> Add/1
  Add/1 -> Data Store Write1/1
  Bit Shift/1 -> Add/2
  word0_msb/1 -> Cast To Single2/1
  [scircv_buffer] -> word0_msb/1
  Constant2/1 -> word0_msb/2
  scircv_buffer/1 -> [scircv_buffer]
  word0_lsb/1 -> Cast To Single1/1
  Constant1/1 -> word0_lsb/2
  [scircv_buffer] -> word0_lsb/1

== system main/Task_Manager/idle/idle_task/comm_npc/comm_npc/COMM_NPC.extractScircv/pri_debug_msgb ==
  note: Note:
      | byte0 - header
      | byte1 - w/r
      | byte2 - func
      | byte3, byte4 - word0_lsb, word0_msb
      | byte5, byte6 - word1_lsb, word1_msb
      | byte7, byte8 - word2_lsb, word2_msb
      | byte9 - chksum
      | byte10 - 0x00
      | byte11 - terminator
  scircv_buffer : Inport
  Action Port : ActionPort  ActionPortLabel=case [ 50 ]:
  Add : Sum  AccumDataTypeStr=uint16  OutDataTypeStr=uint16
  Add1 : Sum  AccumDataTypeStr=uint16  OutDataTypeStr=uint16
  Add2 : Sum  AccumDataTypeStr=uint16  OutDataTypeStr=uint16
  Bit Shift : hdlsllib/Logic and Bit Operations/Bit Shift  mode=Shift Left Logical  N=8
  Bit Shift1 : hdlsllib/Logic and Bit Operations/Bit Shift  mode=Shift Left Logical  N=8
  Bit Shift2 : hdlsllib/Logic and Bit Operations/Bit Shift  mode=Shift Left Logical  N=8
  Cast To Single{1..6} (6 alike) : DataTypeConversion  OutDataTypeStr=uint16  SaturateOnIntegerOverflow=off  RndMeth=Floor
  Constant1 : Constant  Value=3  OutDataTypeStr=uint8
  Constant2 : Constant  Value=4  OutDataTypeStr=uint8
  Constant3 : Constant  Value=7  OutDataTypeStr=uint8
  Constant4 : Constant  Value=8  OutDataTypeStr=uint8
  Constant5 : Constant  Value=5  OutDataTypeStr=uint8
  Constant6 : Constant  Value=6  OutDataTypeStr=uint8
  Data Store Write1 : DataStoreWrite  DataStoreName=debug_msg4  IndexOptions=Index vector (dialog)  Indices=1  OutputSizes=1
  Data Store Write2 : DataStoreWrite  DataStoreName=debug_msg6  IndexOptions=Index vector (dialog)  Indices=1  OutputSizes=1
  Data Store Write3 : DataStoreWrite  DataStoreName=debug_msg5  IndexOptions=Index vector (dialog)  Indices=1  OutputSizes=1
  word0_lsb : Selector  IndexMode=Zero-based  InputPortWidth=12  IndexOptions=Index vector (port)  Indices=[1 3]  OutputSizes=1
  word0_lsb1 : Selector  IndexMode=Zero-based  InputPortWidth=12  IndexOptions=Index vector (port)  Indices=[1 3]  OutputSizes=1
  word0_lsb2 : Selector  IndexMode=Zero-based  InputPortWidth=12  IndexOptions=Index vector (port)  Indices=[1 3]  OutputSizes=1
  word0_msb : Selector  IndexMode=Zero-based  InputPortWidth=12  IndexOptions=Index vector (port)  Indices=[1 3]  OutputSizes=1
  word0_msb1 : Selector  IndexMode=Zero-based  InputPortWidth=12  IndexOptions=Index vector (port)  Indices=[1 3]  OutputSizes=1
  word0_msb2 : Selector  IndexMode=Zero-based  InputPortWidth=12  IndexOptions=Index vector (port)  Indices=[1 3]  OutputSizes=1
  wires:
  [scircv_buffer] -> word0_lsb/1
  Constant1/1 -> word0_lsb/2
  word0_lsb/1 -> Cast To Single1/1
  scircv_buffer/1 -> [scircv_buffer]
  Constant2/1 -> word0_msb/2
  [scircv_buffer] -> word0_msb/1
  word0_msb/1 -> Cast To Single2/1
  Bit Shift/1 -> Add/2
  Add/1 -> Data Store Write1/1
  Cast To Single1/1 -> Add/1
  Cast To Single2/1 -> Bit Shift/1
  Cast To Single4/1 -> Bit Shift1/1
  Cast To Single3/1 -> Add1/1
  Add1/1 -> Data Store Write2/1
  Bit Shift1/1 -> Add1/2
  word0_msb1/1 -> Cast To Single4/1
  [scircv_buffer] -> word0_msb1/1
  Constant4/1 -> word0_msb1/2
  word0_lsb1/1 -> Cast To Single3/1
  Constant3/1 -> word0_lsb1/2
  [scircv_buffer] -> word0_lsb1/1
  Cast To Single6/1 -> Bit Shift2/1
  Cast To Single5/1 -> Add2/1
  Add2/1 -> Data Store Write3/1
  Bit Shift2/1 -> Add2/2
  word0_msb2/1 -> Cast To Single6/1
  [scircv_buffer] -> word0_msb2/1
  Constant6/1 -> word0_msb2/2
  word0_lsb2/1 -> Cast To Single5/1
  Constant5/1 -> word0_lsb2/2
  [scircv_buffer] -> word0_lsb2/1
